simulink model "Controller"  (R2020a)
settings: Solver=FixedStepAuto  StartTime=0.0  StopTime=inf  RelTol=1e-3
model workspace (MAT data in the model file):
  SL_ROS_VariableLengthArrays_MaxSizes.CommonInfo.ArrayTruncateAction = 'EmitWarning'
  SL_ROS_VariableLengthArrays_MaxSizes.MsgTypeMap = containers.Map
  SL_ROS_VariableLengthArrays_MaxSizes.MsgTypeMap.serialization.keys = {'sensor_msgs/CompressedImage', 'sensor_msgs/LaserScan'}
  SL_ROS_VariableLengthArrays_MaxSizes.MsgTypeMap.serialization.values{1}(1).PropertyName = 'Data'
  SL_ROS_VariableLengthArrays_MaxSizes.MsgTypeMap.serialization.values{1}(1).DataType = 'uint8'
  SL_ROS_VariableLengthArrays_MaxSizes.MsgTypeMap.serialization.values{1}(1).MaxLength = 200000
  SL_ROS_VariableLengthArrays_MaxSizes.MsgTypeMap.serialization.values{1}(2).PropertyName = 'Format'
  SL_ROS_VariableLengthArrays_MaxSizes.MsgTypeMap.serialization.values{1}(2).DataType = 'uint8'
  SL_ROS_VariableLengthArrays_MaxSizes.MsgTypeMap.serialization.values{1}(2).MaxLength = 128
  SL_ROS_VariableLengthArrays_MaxSizes.MsgTypeMap.serialization.values{2}(1).PropertyName = 'Intensities'
  SL_ROS_VariableLengthArrays_MaxSizes.MsgTypeMap.serialization.values{2}(1).DataType = 'single'
  SL_ROS_VariableLengthArrays_MaxSizes.MsgTypeMap.serialization.values{2}(1).MaxLength = 360
  SL_ROS_VariableLengthArrays_MaxSizes.MsgTypeMap.serialization.values{2}(2).PropertyName = 'Ranges'
  SL_ROS_VariableLengthArrays_MaxSizes.MsgTypeMap.serialization.values{2}(2).DataType = 'single'
  SL_ROS_VariableLengthArrays_MaxSizes.MsgTypeMap.serialization.values{2}(2).MaxLength = 360
  SL_ROS_VariableLengthArrays_MaxSizes.MsgTypeMap.serialization.uniformity = 0
  SL_ROS_VariableLengthArrays_MaxSizes.MsgTypeMap.serialization.keyType = 'char'
  SL_ROS_VariableLengthArrays_MaxSizes.MsgTypeMap.serialization.valueType = 'any'
values from neighbouring files (symbols this model uses):
  freq = 100    [path_generator.m]
  steering_rate_limit = 100    [path_generator.m]
undefined symbols (not defined in the file or in its folder): Angular, Linear
libraries: robotlib x3, simulink_extras x2, simulink x2, realtime_pacer_lib x2, sharedtransform x1, drivingvehiclecontroller x1
settings Model: Creator=20195009  LastModifiedBy=TruckLabPC2
settings OptimizationCC: EnhancedBackFolding=on  PassReuseOutputArgsAs=Individual arguments  ZeroExternalMemoryAtStartup=off  ZeroInternalMemoryAtStartup=off  MaxStackSize=64  OptimizeBlockOrder=speed  DifferentSizesBufferReuse=on  OptimizationCustomize=off  EfficientTunableParamExpr=on
settings DebuggingCC: ParameterTunabilityLossMsg=error  SFMachineParentedDataDiag=error
settings HardwareCC: ProdBitPerPointer=32  ProdBitPerSizeT=32  ProdBitPerPtrDiffT=32  ProdLargestAtomicFloat=None  ProdIntDivRoundTo=Undefined  ProdEndianess=Unspecified  ProdWordSize=32  ProdHWDeviceType=Generic->Unspecified (assume 32-bit Generic)
settings SFSimCC: MATLABDynamicMemAlloc=off
settings RTWCC: SystemTargetFile=ert.tlc  HardwareBoard=Robot Operating System (ROS)  TemplateMakefile=ert_default_tmf  Toolchain=Catkin  TargetLang=C++
settings CodeAppCC: ForceParamTrailComments=on  IgnoreCustomStorageClasses=off  OperatorAnnotations=on  SimulinkDataObjDesc=on  SFDataObjDesc=on  InsertBlockDesc=on

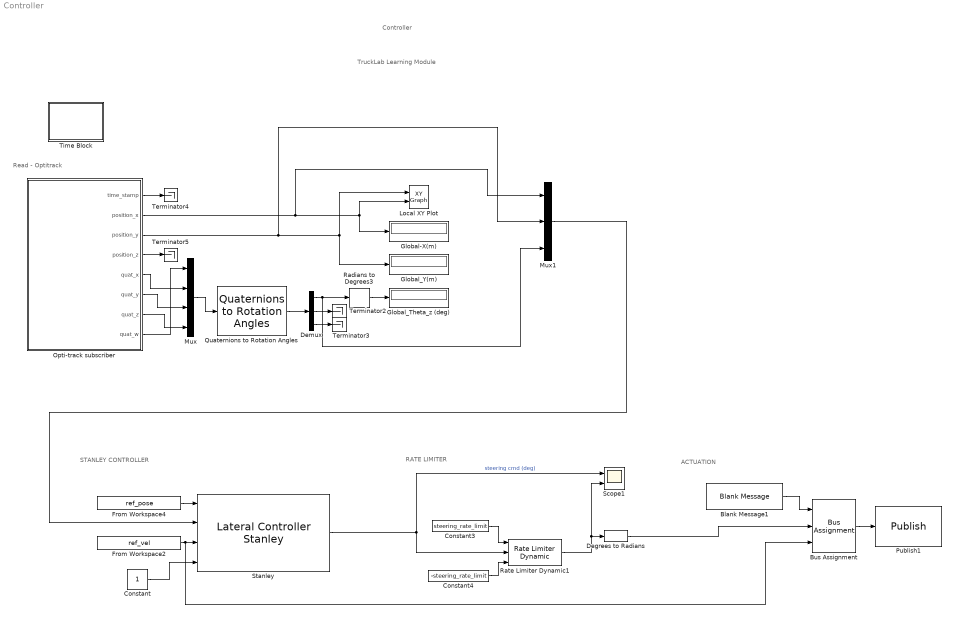
== system Controller ==
  note: ACTUATION
  note: RATE LIMITER
  note: STANLEY CONTROLLER
  note: Read - Optitrack
  note: TruckLab Learning Module
  note: Controller
  Blank Message1 : robotlib/Blank Message  messageClass=Message  entityType=geometry_msgs/Twist  messageType=geometry_msgs/Twist  SampleTime=1/freq
  Bus Assignment : BusAssignment  DialogController=Simulink.DDGSource_BusAssignment  AssignedSignals=Angular.Z,Linear.X
  Constant : Constant
  Constant3 : Constant  Value=steering_rate_limit
  Constant4 : Constant  Value=-steering_rate_limit
  Degrees to Radians : simulink_extras/Transformations/Degrees to Radians
  Demux : Demux  Outputs=3
  From Workspace2 : FromWorkspace  VariableName=ref_vel
  From Workspace4 : FromWorkspace  VariableName=ref_pose
  Global-X(m) : Display
  Global_Theta_z (deg) : Display
  Global_Y(m) : Display
  Local XY Plot : simulink/Sinks/XY Graph  xmin=0  xmax=6  ymin=0  ymax=6  st=-1
  Mux : Mux
  Mux1 : Mux  Inputs=3
  Opti-track subscriber : Subsystem
  Publish1 : robotlib/Publish  topicSource=Specify your own  topic=/tractor1/cmd_tractor1  messageType=geometry_msgs/Twist  messageQueueLength=1
      link override SinkBlock: ROSTopic=/cmd_vel  ROSMessageType=geometry_msgs/Twist  SLBusName=SL_Bus_TruckLab_MannualDrivingROS1_geometry_msgs_Twist  ModelName=TruckLab_MannualDrivingROS1  BlockId=Pub_TruckLab_MannualDrivingROS1_402
  Quaternions to Rotation Angles : sharedtransform/Quaternions to Rotation Angles  rotationOrder=ZXY  aMode=aMode
      settings: SourceProductBaseCode=AE,PW,MT,VE,VP
  Radians to Degrees3 : simulink_extras/Transformations/Radians to Degrees
  Rate Limiter Dynamic1 : simulink/Discontinuities/Rate Limiter Dynamic
  Scope1 : Scope  NumInputPorts=2
  Stanley : drivingvehiclecontroller/Lateral Controller Stanley  ModelType=Kinematic bicycle model  PositionGainF=ref_Kf  PositionGainR=ref_Kr  YawRateGain=0.2  DelayGain=0.2  VehicleMass=1575  Lf=1.2  Lr=1.6  TireStiffness=19000  Wheelbase=0.272  MaxSteeringAngle=25
      settings: SourceProductBaseCode=DR
  Terminator{2..5} (4 alike) : Terminator
  Time Block : Subsystem
  wires:
  Opti-track subscriber/3(position_y) -> Global_Y(m)/1, Local XY Plot/1, Mux1/2
  Opti-track subscriber/2(position_x) -> Mux1/1, Global-X(m)/1, Local XY Plot/2
  Mux/1 -> Quaternions to Rotation Angles/1
  Quaternions to Rotation Angles/1 -> Demux/1
  Demux/1 -> Mux1/3, Radians to Degrees3/1
  Radians to Degrees3/1 -> Global_Theta_z (deg)/1
  Demux/2 -> Terminator2/1
  Demux/3 -> Terminator3/1
  Opti-track subscriber/5(quat_x) -> Mux/2
  Opti-track subscriber/6(quat_y) -> Mux/3
  Opti-track subscriber/7(quat_z) -> Mux/4
  Opti-track subscriber/8(quat_w) -> Mux/1
  Opti-track subscriber/1(time_stamp) -> Terminator4/1
  Opti-track subscriber/4(position_z) -> Terminator5/1
  Constant/1 -> Stanley/4
  From Workspace4/1 -> Stanley/1
  Mux1/1 -> Stanley/2
  Stanley/1 -> Rate Limiter Dynamic1/2, Scope1/1  "steering cmd (deg)"
  From Workspace2/1 -> Bus Assignment/3, Stanley/3
  Blank Message1/1 -> Bus Assignment/1
  Bus Assignment/1 -> Publish1/1
  Degrees to Radians/1 -> Bus Assignment/2
  Constant4/1 -> Rate Limiter Dynamic1/3
  Constant3/1 -> Rate Limiter Dynamic1/1
  Rate Limiter Dynamic1/1 -> Scope1/2, Degrees to Radians/1

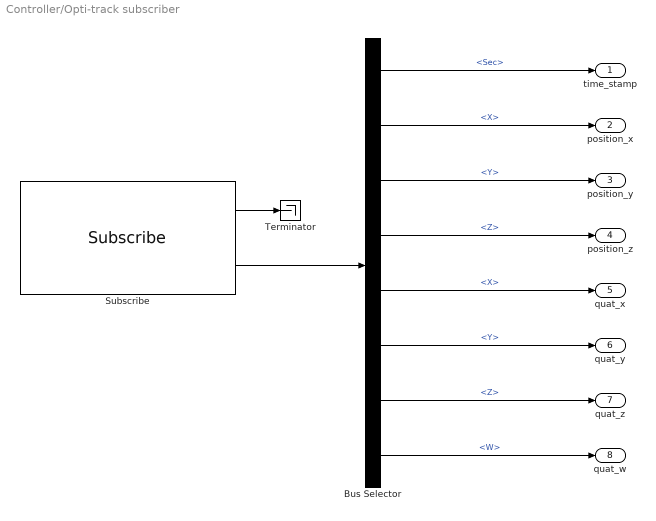
== system Controller/Opti-track subscriber ==
  Bus Selector : BusSelector  OutputSignals=Header.Stamp.Sec,Pose.Position.X,Pose.Position.Y,Pose.Position.Z,Pose.Orientation.X,Pose.Orientation.Y,Pose.Orientation.Z,Pose.Orientation.W
  Subscribe : robotlib/Subscribe  topicSource=Select from ROS network  topic=/DC_1/TRACTOR_1/optitrack  messageType=geometry_msgs/PoseStamped  sampleTime=-1  messageQueueLength=1
  Terminator : Terminator
  time_stamp : Outport
  position_x : Outport  Port=2
  position_y : Outport  Port=3
  position_z : Outport  Port=4
  quat_x : Outport  Port=5
  quat_y : Outport  Port=6
  quat_z : Outport  Port=7
  quat_w : Outport  Port=8
  wires:
  Subscribe/1 -> Terminator/1
  Subscribe/2 -> Bus Selector/1
  Bus Selector/1 -> time_stamp/1  "<Sec>"
  Bus Selector/2 -> position_x/1  "<X>"
  Bus Selector/3 -> position_y/1  "<Y>"
  Bus Selector/4 -> position_z/1  "<Z>"
  Bus Selector/5 -> quat_x/1  "<X>"
  Bus Selector/6 -> quat_y/1  "<Y>"
  Bus Selector/7 -> quat_z/1  "<Z>"
  Bus Selector/8 -> quat_w/1  "<W>"

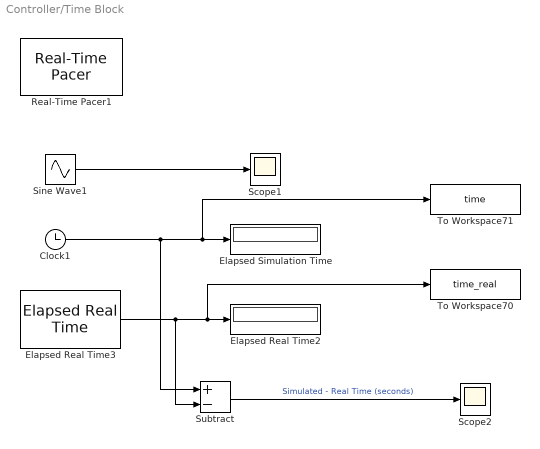
== system Controller/Time Block ==
  Clock1 : Clock
  Elapsed Real Time2 : Display
      settings: Decimation=2
  Elapsed Real Time3 : realtime_pacer_lib/Elapsed Real Time
  Elapsed Simulation Time : Display
      settings: Decimation=2
  Real-Time Pacer1 : realtime_pacer_lib/Real-Time Pacer  simTimePerRealTime=1
  Scope1 : Scope
  Scope2 : Scope
  Sine Wave1 : Sin  Frequency=2*pi*0.5  SampleTime=0
  Subtract : Sum  Inputs=+-
  To Workspace70 : ToWorkspace  VariableName=time_real  SampleTime=-1
  To Workspace71 : ToWorkspace  VariableName=time  SampleTime=-1
  wires:
  Subtract/1 -> Scope2/1  "Simulated - Real Time (seconds)"
  Elapsed Real Time3/1 -> Elapsed Real Time2/1, To Workspace70/1, Subtract/2
  Sine Wave1/1 -> Scope1/1
  Clock1/1 -> Subtract/1, Elapsed Simulation Time/1, To Workspace71/1
